simulink model "Kp_Effect"  (R2024b)
settings: Solver=FixedStepAuto  StartTime=0.0  StopTime=13  FixedStep=0.0001  RelTol=1e-3  EnableMultiTasking=on
libraries: arduinolib x2
settings Model: ExtModeTrigDuration=2  Creator=abdal  LastModifiedBy=abdal
settings SolverCC: AutoInsertRateTranBlk=on
settings OptimizationCC: EnhancedBackFolding=on  PassReuseOutputArgsAs=Individual arguments  ZeroExternalMemoryAtStartup=off  ZeroInternalMemoryAtStartup=off  MaxStackSize=64  OptimizeBlockOrder=speed  DifferentSizesBufferReuse=on  OptimizationCustomize=off  EfficientTunableParamExpr=on
settings DebuggingCC: ParameterTunabilityLossMsg=error
settings HardwareCC: ProdBitPerInt=16  ProdBitPerPointer=16  ProdBitPerSizeT=16  ProdBitPerPtrDiffT=16  ProdLargestAtomicFloat=None  ProdWordSize=8  ProdHWDeviceType=Atmel->AVR
settings SFSimCC: MATLABDynamicMemAlloc=off
settings RTWCC: Description=Embedded Coder  SystemTargetFile=ert.tlc  HardwareBoard=Arduino Uno  TemplateMakefile=ert_default_tmf  Toolchain=Arduino AVR  BuildConfiguration=Faster Runs
settings CodeAppCC: ForceParamTrailComments=on  IgnoreCustomStorageClasses=off  OperatorAnnotations=on  SimulinkDataObjDesc=on  SFDataObjDesc=on  InsertBlockDesc=on
settings ERTTargetCC: SupportContinuousTime=on  SupportVariableSizeSignals=on  ExtModeTransport=3  ExtModeStaticAlloc=on  ExtModeAutomaticAllocSize=off  ExtModeStaticAllocSize=250  ExtModeMexFile=ext_xcp  ExtModeIntrfLevel=Level2 - Open  InlinedParameterPlacement=Hierarchical

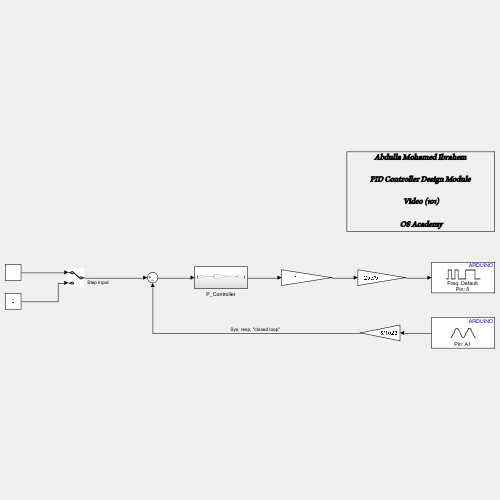
[thumbnail: Simulink's stored preview of the top-level diagram]
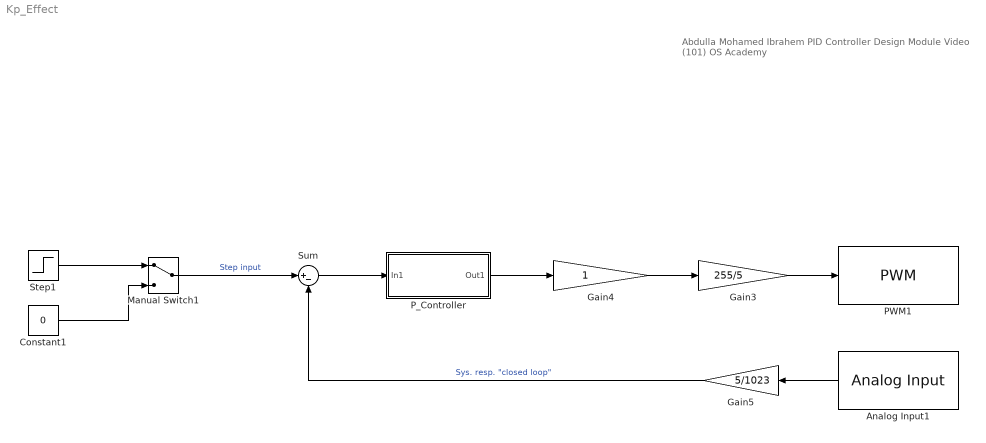
== system Kp_Effect ==
  note: Abdulla Mohamed Ibrahem
      | PID Controller Design Module
      | Video (101)
      | OS Academy
  Analog Input1 : arduinolib/Analog Input  pinNumber=1  ReadResultsOnly=off  ConversionTriggerSource=Software  ExternalTriggerType=uint32( 0 )  OutputDataType=uint16  EnableConversionCompleteNotify=off  EnableOuputStatus=off  SampleTime=-1  blockPlatform=arduino
  Constant1 : Constant  Value=0
  Gain3 : Gain  Gain=255/5
  Gain4 : Gain
  Gain5 : Gain  Gain=5/1023
  Manual Switch1 : ManualSwitch
  PWM1 : arduinolib/PWM  pinNumber=5  frequencyType=Default  desiredFrequency=490.2  achievableFrequency=490.2
  P_Controller : Subsystem
  Step1 : Step  Time=2  SampleTime=0
  Sum : Sum  Inputs=|+-
  wires:
  Gain3/1 -> PWM1/1
  Sum/1 -> P_Controller/1(In1)
  Gain4/1 -> Gain3/1
  Analog Input1/1 -> Gain5/1
  Gain5/1 -> Sum/2  "Sys. resp. \"closed loop\""
  Step1/1 -> Manual Switch1/1
  Constant1/1 -> Manual Switch1/2
  Manual Switch1/1 -> Sum/1  "Step input"
  P_Controller/1(Out1) -> Gain4/1

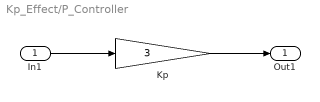
== system Kp_Effect/P_Controller ==
  In1 : Inport
  Kp : Gain  Gain=3
  Out1 : Outport
  wires:
  In1/1 -> Kp/1
  Kp/1 -> Out1/1
